simulink model "vc_coder"  (R2019b)
settings: Solver=FixedStepDiscrete  StartTime=0.0  StopTime=Inf  FixedStep=0.025  RelTol=1e-3  EnableMultiTasking=on
PreLoadFcn:
  | mdlname = bdroot;
  | oldFolder = cd(fileparts(which(mdlname)));
  | % cd ..\
  | 
  | load('./bus_type/bus_type.mat');
model workspace (MAT data in the model file):
  CLK = Simulink.Parameter
  CLK.Value = 200000000
  CLK.DataType = 'auto'
  CLK.Dimensions = [1 1]
  PWMFreq = Simulink.Parameter
  PWMFreq.Value = 1200
  PWMFreq.DataType = 'auto'
  PWMFreq.Dimensions = [1 1]
  RCDataLen = Simulink.Parameter
  RCDataLen.Value = 19
  RCDataLen.DataType = 'int8'
  RCDataLen.Dimensions = [1 1]
  StepSize = Simulink.Parameter
  StepSize.Value = 0.025
  StepSize.DataType = 'auto'
  StepSize.Dimensions = [1 1]
libraries: c2837xDlib x9, simulink x5, c280xlib x2, commutil2 x1, c2000lib x1
CloseFcn:
  | cd(oldFolder);
Description:
  | -> System Description <-
  | - Development environment:
  |     Matlab (version 2019b) with licence to
  |     - Simulink
  |     - Embedded Coder Support Package for Texas Instruments C2000 Processors
  |     - StateFlow
  | - Control board:
  |     TI LAUNCHXL F28379D
settings Model: SimulationMode=external  ExtModeTrigDuration=8  OrderedModelArguments=off  Creator=Quinn Ding  LastModifiedBy=Quinn
settings OptimizationCC: DefaultUnderspecifiedDataType=single  EnhancedBackFolding=on  PassReuseOutputArgsAs=Individual arguments  ZeroExternalMemoryAtStartup=off  MaxStackSize=1024  OptimizeBlockOrder=speed  DifferentSizesBufferReuse=on  OptimizationCustomize=off  DenormalBehavior=FlushToZero  EfficientTunableParamExpr=on
settings DebuggingCC: ParameterTunabilityLossMsg=error
settings HardwareCC: ProdBitPerChar=16  ProdBitPerInt=16  ProdBitPerPointer=32  ProdBitPerSizeT=32  ProdBitPerPtrDiffT=32  ProdLargestAtomicInteger=Integer  ProdLargestAtomicFloat=None  ProdWordSize=16  ProdLongLongMode=on  ProdHWDeviceType=Texas Instruments->C2000
settings SFSimCC: MATLABDynamicMemAlloc=off
settings RTWCC: SystemTargetFile=ert.tlc  HardwareBoard=TI Delfino F28379D LaunchPad  TLCOptions=-aInlineSetEventsForThisBaseRateFcn=TLC_FALSE -aSuppressMultiTaskScheduler=TLC_FALSE -aRateBasedStepFcn=1  TemplateMakefile=ert_default_tmf  Toolchain=Texas Instruments Code Composer Studio (C2000)  BuildConfiguration=Faster Runs  IncludeHyperlinkInReport=on
settings CodeAppCC: ForceParamTrailComments=on  IgnoreCustomStorageClasses=off  OperatorAnnotations=on  SimulinkDataObjDesc=on  SFDataObjDesc=on  InsertBlockDesc=on
settings ERTTargetCC: TargetLangStandard=C99 (ISO)  CodeReplacementLibrary=TI C28x  ExtModeStaticAllocSize=10000  RootIOFormat=Structure reference

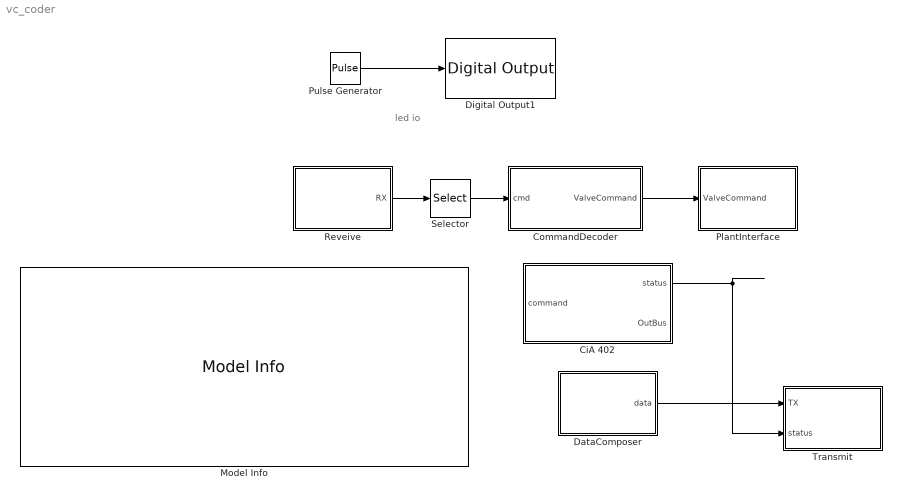
== system vc_coder ==
  note: led io
  CiA 402 : Stateflow chart  BlockKeywords=__PRM__SERIALIZED__DATA__:Stateflow Chart,Stateflow Diagram  TreatAsAtomicUnit=on
  CommandDecoder : Subsystem
  DataComposer : Subsystem
  Digital Output1 : c2837xDlib/Digital Output  GPIO_Number=GPIO24~GPIO31  GPIO_Bit0=off  GPIO_BIT0_Toggle=off  GPIO_Bit1=off  GPIO_BIT1_Toggle=off  GPIO_Bit2=off  GPIO_BIT2_Toggle=off  GPIO_Bit3=off  GPIO_BIT3_Toggle=off  GPIO_Bit4=off  GPIO_BIT4_Toggle=off  GPIO_Bit5=off  GPIO_BIT5_Toggle=off  GPIO_Bit6=off  GPIO_BIT6_Toggle=off  GPIO_Bit7=on  GPIO_BIT7_Toggle=off
      settings: SourceProductName=Embedded Coder Support Package for Texas Instruments C2000 Processors  SourceProductBaseCode=TIC2000
  Model Info : simulink/Model-Wide Utilities/Model Info  Frame=on  DisplayStringWithTags=|  HorizontalTextAlignment=Left  LeftAlignmentValue=0.02
      | DSP coder %<ModelVersion> of valve controller for the SMA actuator.
      | 
      | Developed by %<Creator> at the Surgical Robotics & Devices Laboratory, CUHK.
      | 
      | Last updated at %<LastModificationDate>.
      | 
      | %<Description>
  PlantInterface : Subsystem
  Pulse Generator : DiscretePulseGenerator  Period=100  PulseWidth=50  SampleTime=-1
  Reveive : Subsystem
  Selector : Selector  InputPortWidth=19  IndexOptions=Index vector (dialog)  Indices=[RCDataLen]  OutputSizes=1
  Transmit : Subsystem
  wires:
  Pulse Generator/1 -> Digital Output1/1
  CommandDecoder/1(ValveCommand) -> PlantInterface/1(ValveCommand)
  Reveive/1(RX) -> Selector/1
  DataComposer/1(data) -> Transmit/1(TX)
  CiA 402/1(status) -> Transmit/2(status)
  Selector/1 -> CommandDecoder/1(cmd)

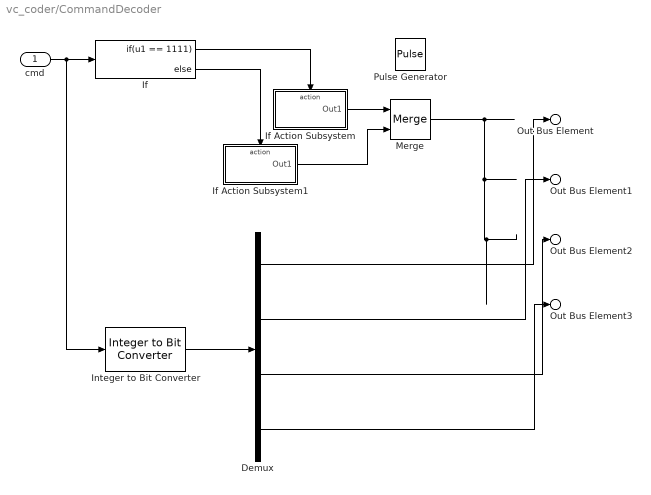
== system vc_coder/CommandDecoder ==
  cmd : Inport
  Demux : Demux
  If : If  IfExpression=u1 == 1111
  If Action Subsystem : Subsystem  TreatAsAtomicUnit=on
  If Action Subsystem1 : Subsystem  TreatAsAtomicUnit=on
  Integer to Bit Converter : commutil2/Integer to Bit Converter  nbits=4  signedInputValues=Unsigned  bitOrder=MSB first  outDtype=Inherit via internal rule
      settings: SourceProductName=Communications Toolbox
  Merge : Merge
  Pulse Generator : DiscretePulseGenerator  Period=80  PulseWidth=40  SampleTime=-1
  Out Bus Element : Outport  PortName=ValveCommand  Element=V1
  Out Bus Element1 : Outport  PortName=ValveCommand  Element=V2
  Out Bus Element2 : Outport  PortName=ValveCommand  Element=V3
  Out Bus Element3 : Outport  PortName=ValveCommand  Element=V4
  wires:
  Merge/1 -> ?
  If/1 -> If Action Subsystem/Action
  If/2 -> If Action Subsystem1/Action
  If Action Subsystem/1(Out1) -> Merge/1
  If Action Subsystem1/1(Out1) -> Merge/2
  cmd/1 -> Integer to Bit Converter/1, If/1
  Integer to Bit Converter/1 -> Demux/1
  Demux/1 -> Out Bus Element/1
  Demux/2 -> Out Bus Element1/1
  Demux/3 -> Out Bus Element2/1
  Demux/4 -> Out Bus Element3/1

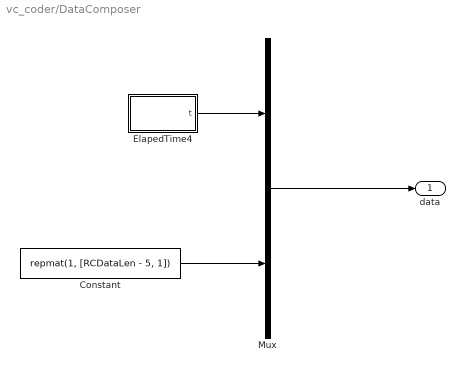
== system vc_coder/DataComposer ==
  Constant : Constant  Value=repmat(1, [RCDataLen - 5, 1])  OutDataTypeStr=single
  ElapedTime4 : Subsystem
  Mux : Mux  Inputs=2
  data : Outport
  wires:
  ElapedTime4/1(t) -> Mux/1
  Mux/1 -> data/1
  Constant/1 -> Mux/2

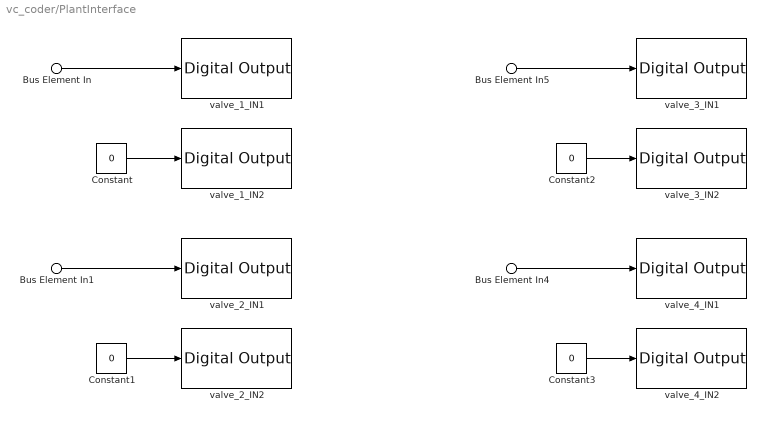
== system vc_coder/PlantInterface ==
  Bus Element In1 : Inport  PortName=ValveCommand  Element=V2
  Bus Element In : Inport  PortName=ValveCommand  Element=V1
  Bus Element In5 : Inport  PortName=ValveCommand  Element=V3
  Bus Element In4 : Inport  PortName=ValveCommand  Element=V4
  Constant{,1..3} (4 alike) : Constant  Value=0
  valve_1_IN1 : c2837xDlib/Digital Output  GPIO_Number=GPIO0~GPIO7  GPIO_Bit0=off  GPIO_BIT0_Toggle=off  GPIO_Bit1=off  GPIO_BIT1_Toggle=off  GPIO_Bit2=off  GPIO_BIT2_Toggle=off  GPIO_Bit3=off  GPIO_BIT3_Toggle=off  GPIO_Bit4=off  GPIO_BIT4_Toggle=off  GPIO_Bit5=off  GPIO_BIT5_Toggle=off  GPIO_Bit6=on  GPIO_BIT6_Toggle=off  GPIO_Bit7=off  GPIO_BIT7_Toggle=off
      settings: SourceProductName=Embedded Coder Support Package for Texas Instruments C2000 Processors  SourceProductBaseCode=TIC2000
  valve_1_IN2 : c2837xDlib/Digital Output  GPIO_Number=GPIO0~GPIO7  GPIO_Bit0=off  GPIO_BIT0_Toggle=off  GPIO_Bit1=off  GPIO_BIT1_Toggle=off  GPIO_Bit2=off  GPIO_BIT2_Toggle=off  GPIO_Bit3=off  GPIO_BIT3_Toggle=off  GPIO_Bit4=off  GPIO_BIT4_Toggle=off  GPIO_Bit5=off  GPIO_BIT5_Toggle=off  GPIO_Bit6=off  GPIO_BIT6_Toggle=off  GPIO_Bit7=on  GPIO_BIT7_Toggle=off
      settings: SourceProductName=Embedded Coder Support Package for Texas Instruments C2000 Processors  SourceProductBaseCode=TIC2000
  valve_2_IN1 : c2837xDlib/Digital Output  GPIO_Number=GPIO8~GPIO15  GPIO_Bit0=on  GPIO_BIT0_Toggle=off  GPIO_Bit1=off  GPIO_BIT1_Toggle=off  GPIO_Bit2=off  GPIO_BIT2_Toggle=off  GPIO_Bit3=off  GPIO_BIT3_Toggle=off  GPIO_Bit4=off  GPIO_BIT4_Toggle=off  GPIO_Bit5=off  GPIO_BIT5_Toggle=off  GPIO_Bit6=off  GPIO_BIT6_Toggle=off  GPIO_Bit7=off  GPIO_BIT7_Toggle=off
      settings: SourceProductName=Embedded Coder Support Package for Texas Instruments C2000 Processors  SourceProductBaseCode=TIC2000
  valve_2_IN2 : c2837xDlib/Digital Output  GPIO_Number=GPIO8~GPIO15  GPIO_Bit0=off  GPIO_BIT0_Toggle=off  GPIO_Bit1=on  GPIO_BIT1_Toggle=off  GPIO_Bit2=off  GPIO_BIT2_Toggle=off  GPIO_Bit3=off  GPIO_BIT3_Toggle=off  GPIO_Bit4=off  GPIO_BIT4_Toggle=off  GPIO_Bit5=off  GPIO_BIT5_Toggle=off  GPIO_Bit6=off  GPIO_BIT6_Toggle=off  GPIO_Bit7=off  GPIO_BIT7_Toggle=off
      settings: SourceProductName=Embedded Coder Support Package for Texas Instruments C2000 Processors  SourceProductBaseCode=TIC2000
  valve_3_IN1 : c2837xDlib/Digital Output  GPIO_Number=GPIO0~GPIO7  GPIO_Bit0=off  GPIO_BIT0_Toggle=off  GPIO_Bit1=off  GPIO_BIT1_Toggle=off  GPIO_Bit2=off  GPIO_BIT2_Toggle=off  GPIO_Bit3=off  GPIO_BIT3_Toggle=off  GPIO_Bit4=on  GPIO_BIT4_Toggle=off  GPIO_Bit5=off  GPIO_BIT5_Toggle=off  GPIO_Bit6=off  GPIO_BIT6_Toggle=off  GPIO_Bit7=off  GPIO_BIT7_Toggle=off
      settings: SourceProductName=Embedded Coder Support Package for Texas Instruments C2000 Processors  SourceProductBaseCode=TIC2000
  valve_3_IN2 : c2837xDlib/Digital Output  GPIO_Number=GPIO0~GPIO7  GPIO_Bit0=off  GPIO_BIT0_Toggle=off  GPIO_Bit1=off  GPIO_BIT1_Toggle=off  GPIO_Bit2=off  GPIO_BIT2_Toggle=off  GPIO_Bit3=off  GPIO_BIT3_Toggle=off  GPIO_Bit4=off  GPIO_BIT4_Toggle=off  GPIO_Bit5=on  GPIO_BIT5_Toggle=off  GPIO_Bit6=off  GPIO_BIT6_Toggle=off  GPIO_Bit7=off  GPIO_BIT7_Toggle=off
      settings: SourceProductName=Embedded Coder Support Package for Texas Instruments C2000 Processors  SourceProductBaseCode=TIC2000
  valve_4_IN1 : c2837xDlib/Digital Output  GPIO_Number=GPIO8~GPIO15  GPIO_Bit0=off  GPIO_BIT0_Toggle=off  GPIO_Bit1=off  GPIO_BIT1_Toggle=off  GPIO_Bit2=on  GPIO_BIT2_Toggle=off  GPIO_Bit3=off  GPIO_BIT3_Toggle=off  GPIO_Bit4=off  GPIO_BIT4_Toggle=off  GPIO_Bit5=off  GPIO_BIT5_Toggle=off  GPIO_Bit6=off  GPIO_BIT6_Toggle=off  GPIO_Bit7=off  GPIO_BIT7_Toggle=off
      settings: SourceProductName=Embedded Coder Support Package for Texas Instruments C2000 Processors  SourceProductBaseCode=TIC2000
  valve_4_IN2 : c2837xDlib/Digital Output  GPIO_Number=GPIO8~GPIO15  GPIO_Bit0=off  GPIO_BIT0_Toggle=off  GPIO_Bit1=off  GPIO_BIT1_Toggle=off  GPIO_Bit2=off  GPIO_BIT2_Toggle=off  GPIO_Bit3=on  GPIO_BIT3_Toggle=off  GPIO_Bit4=off  GPIO_BIT4_Toggle=off  GPIO_Bit5=off  GPIO_BIT5_Toggle=off  GPIO_Bit6=off  GPIO_BIT6_Toggle=off  GPIO_Bit7=off  GPIO_BIT7_Toggle=off
      settings: SourceProductName=Embedded Coder Support Package for Texas Instruments C2000 Processors  SourceProductBaseCode=TIC2000
  wires:
  Constant1/1 -> valve_2_IN2/1
  Bus Element In1/1 -> valve_2_IN1/1
  Constant/1 -> valve_1_IN2/1
  Bus Element In/1 -> valve_1_IN1/1
  Bus Element In5/1 -> valve_3_IN1/1
  Bus Element In4/1 -> valve_4_IN1/1
  Constant3/1 -> valve_4_IN2/1
  Constant2/1 -> valve_3_IN2/1

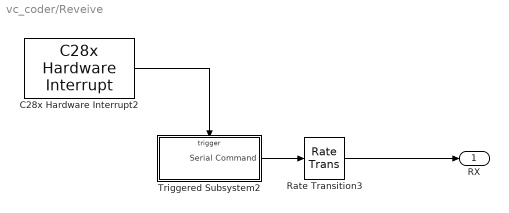
== system vc_coder/Reveive ==
  C28x Hardware Interrupt2 : c2000lib/Scheduling/C28x Hardware Interrupt  irqnumbers=[9]  pienumbers=[3]  irqpriorities=[30]  irqpreempts=[0]  showinput=off  dspchiptype=C280X
      settings: SourceProductName=Embedded Coder Support Package for Texas Instruments C2000 Processors  SourceProductBaseCode=TIC2000
  Rate Transition3 : RateTransition  Deterministic=off  OutPortSampleTimeOpt=Inherit
  Triggered Subsystem2 : Subsystem  TreatAsAtomicUnit=on
  RX : Outport
  wires:
  C28x Hardware Interrupt2/1 -> Triggered Subsystem2/Trigger
  Triggered Subsystem2/1(Serial Command) -> Rate Transition3/1
  Rate Transition3/1 -> RX/1

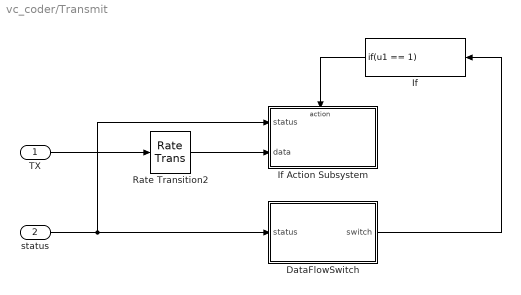
== system vc_coder/Transmit ==
  TX : Inport
  status : Inport  Port=2
  DataFlowSwitch : Subsystem
  If : If  IfExpression=u1 == 1  ShowElse=off
  If Action Subsystem : Subsystem  TreatAsAtomicUnit=on
  Rate Transition2 : RateTransition  Deterministic=off
  wires:
  If/1 -> If Action Subsystem/Action
  Rate Transition2/1 -> If Action Subsystem/2(data)
  TX/1 -> Rate Transition2/1
  status/1 -> If Action Subsystem/1(status), DataFlowSwitch/1(status)
  DataFlowSwitch/1(switch) -> If/1

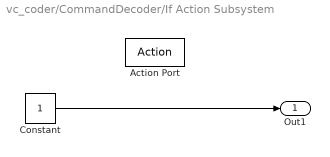
== system vc_coder/CommandDecoder/If Action Subsystem ==
  Action Port : ActionPort  ActionPortLabel=if(u1 == 1111)
  Constant : Constant
  Out1 : Outport
  wires:
  Constant/1 -> Out1/1

== system vc_coder/CommandDecoder/If Action Subsystem1 ==
  Action Port : ActionPort  ActionPortLabel=else
  Constant : Constant  Value=0
  Out1 : Outport
  wires:
  Constant/1 -> Out1/1

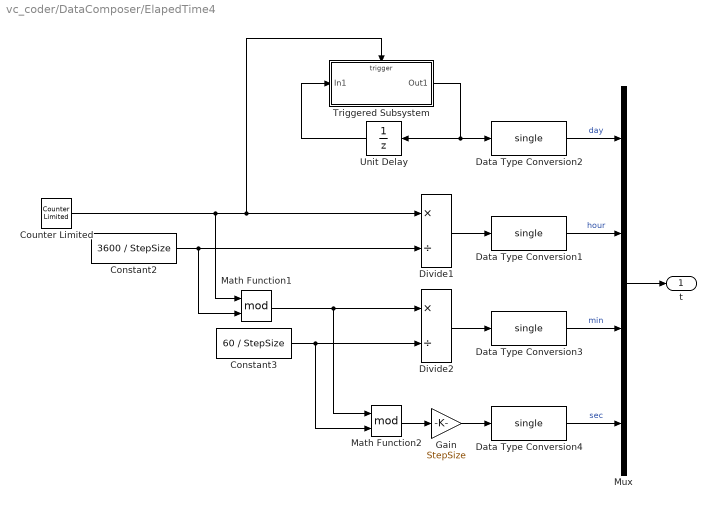
== system vc_coder/DataComposer/ElapedTime4 ==
  Constant2 : Constant  Value=3600 / StepSize  OutDataTypeStr=uint32
  Constant3 : Constant  Value=60 / StepSize  OutDataTypeStr=uint32
  Counter Limited : simulink/Sources/Counter Limited  uplimit=1 / StepSize * 60 * 60 * 24  tsamp=-1
  Data Type Conversion{1..4} (4 alike) : DataTypeConversion  OutDataTypeStr=single
  Divide1 : Product  Inputs=*/  OutDataTypeStr=uint8
  Divide2 : Product  Inputs=*/  OutDataTypeStr=uint8
  Gain : Gain  Gain=StepSize  OutDataTypeStr=single
  Math Function1 : Math  Operator=mod  SignedPower=off  SaturateOnIntegerOverflow=on
  Math Function2 : Math  Operator=mod  SignedPower=off  SaturateOnIntegerOverflow=on
  Mux : Mux
  Triggered Subsystem : Subsystem  TreatAsAtomicUnit=on
  Unit Delay : UnitDelay  SampleTime=-1  HasFrameUpgradeWarning=on
  t : Outport
  wires:
  Counter Limited/1 -> Divide1/1, Triggered Subsystem/Trigger, Math Function1/1
  Divide1/1 -> Data Type Conversion1/1
  Divide2/1 -> Data Type Conversion3/1
  Constant2/1 -> Math Function1/2, Divide1/2
  Math Function1/1 -> Divide2/1, Math Function2/1
  Data Type Conversion2/1 -> Mux/1  "day"
  Data Type Conversion1/1 -> Mux/2  "hour"
  Data Type Conversion3/1 -> Mux/3  "min"
  Data Type Conversion4/1 -> Mux/4  "sec"
  Math Function2/1 -> Gain/1
  Constant3/1 -> Divide2/2, Math Function2/2
  Mux/1 -> t/1
  Triggered Subsystem/1(Out1) -> Data Type Conversion2/1, Unit Delay/1
  Unit Delay/1 -> Triggered Subsystem/1(In1)
  Gain/1 -> Data Type Conversion4/1

== system vc_coder/Reveive/Triggered Subsystem2 ==
  SCIA RCV Interrupt : TriggerPort  TriggerType=function-call  VariantControl=Variant
  SCI Receive : c280xlib/SCI Receive  sciModule=B  dataHead=''  dataTail=''  dataType=single  dataDim=19  initValue=0  errOption=Output the last received value  errValue=0  sampleTime=-1  outputStatus=off  postInterrupt=on  numFifo=1
      settings: SourceProductName=Embedded Coder Support Package for Texas Instruments C2000 Processors  SourceProductBaseCode=TIC2000
  Serial Command : Outport
  wires:
  SCI Receive/1 -> Serial Command/1

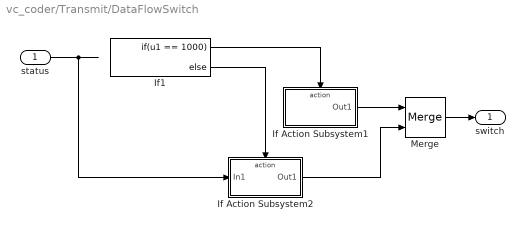
== system vc_coder/Transmit/DataFlowSwitch ==
  status : Inport
  If Action Subsystem1 : Subsystem  TreatAsAtomicUnit=on
  If Action Subsystem2 : Subsystem  TreatAsAtomicUnit=on
  If1 : If  IfExpression=u1 == 1000
  Merge : Merge
  switch : Outport
  wires:
  If Action Subsystem1/1(Out1) -> Merge/1
  If Action Subsystem2/1(Out1) -> Merge/2
  If1/2 -> If Action Subsystem2/Action
  Merge/1 -> switch/1
  If1/1 -> If Action Subsystem1/Action
  status/1 -> If Action Subsystem2/1(In1)

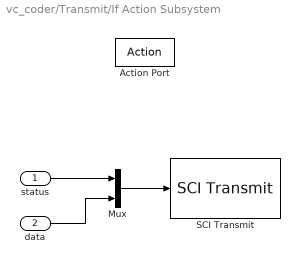
== system vc_coder/Transmit/If Action Subsystem ==
  status : Inport
  data : Inport  Port=2
  Action Port : ActionPort  ActionPortLabel=if(u1 == 1)
  Mux : Mux  Inputs=2
  SCI Transmit : c280xlib/SCI Transmit  sciModule=B  dataHead=''  dataTail=''  postInterrupt=off  numFifo=1
      settings: SourceProductName=Embedded Coder Support Package for Texas Instruments C2000 Processors
  wires:
  status/1 -> Mux/1
  data/1 -> Mux/2
  Mux/1 -> SCI Transmit/1

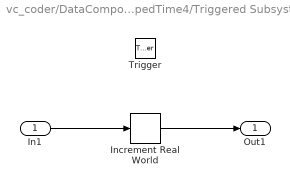
== system vc_coder/DataComposer/ElapedTime4/Triggered Subsystem ==
  In1 : Inport
  Trigger : TriggerPort  TriggerType=falling  VariantControl=Variant
  Increment Real World : simulink/Additional Math & Discrete/Additional Math: Increment - Decrement/Increment Real World
      settings: SourceProductName=Simulink  SourceProductBaseCode=SL
  Out1 : Outport
  wires:
  In1/1 -> Increment Real World/1
  Increment Real World/1 -> Out1/1

== system vc_coder/Transmit/DataFlowSwitch/If Action Subsystem1 ==
  Action Port : ActionPort  ActionPortLabel=if(u1 == 1000)
  Constant : Constant
  Out1 : Outport
  wires:
  Constant/1 -> Out1/1

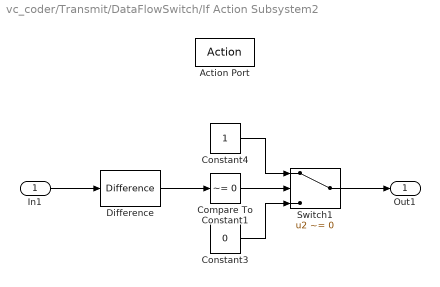
== system vc_coder/Transmit/DataFlowSwitch/If Action Subsystem2 ==
  In1 : Inport
  Action Port : ActionPort  ActionPortLabel=else
  Compare To Constant1 : simulink/Logic and Bit Operations/Compare To Constant  relop=~=  const=0  OutDataTypeStr=boolean
  Constant3 : Constant  Value=0
  Constant4 : Constant
  Difference : simulink/Discrete/Difference  ICPrevInput=0.0  OutMin=[]  OutMax=[]  OutDataType=fixdt(1, 16)  OutScaling=2^-10  DoSatur=off
  Switch1 : Switch  Criteria=u2 ~= 0
  Out1 : Outport
  wires:
  Switch1/1 -> Out1/1
  Compare To Constant1/1 -> Switch1/2
  In1/1 -> Difference/1
  Constant3/1 -> Switch1/3
  Difference/1 -> Compare To Constant1/1
  Constant4/1 -> Switch1/1

== stateflow chart vc_coder/CiA 402 ==
  state READY_TO_SWITCH_ON
    entry:
    status = 50;
    exit:
    ;
  state SWITCHED_ON
    entry:
    OutBus.EnableValve1 = 0;
    OutBus.EnableValve2 = 0;
    status = 51;
    exit:
    ;
  state OPERATION_ENABLE
    entry:
    OutBus.EnableValve1 = 1;
    OutBus.EnableValve2 = 1;
    status = 52;
    exit:
    ;
    state IDLE_MODE
      entry:
      status = 52;
    state PRECOOL_MODE
      entry:
      status = 53;
    (default) -> IDLE_MODE
    IDLE_MODE -> PRECOOL_MODE : [command(RCDataLen) == 14]
    PRECOOL_MODE -> IDLE_MODE : [command(RCDataLen) == 15]
  OPERATION_ENABLE -> READY_TO_SWITCH_ON [order 2] : [command(RCDataLen) == 0]
  SWITCHED_ON -> READY_TO_SWITCH_ON [order 3] : [command(RCDataLen) == 0]
  (default) -> READY_TO_SWITCH_ON
  SWITCHED_ON -> OPERATION_ENABLE [order 2] : [command(RCDataLen) == 12]
  READY_TO_SWITCH_ON -> SWITCHED_ON : [command(RCDataLen) == 10]
  SWITCHED_ON -> READY_TO_SWITCH_ON [order 1] : [command(RCDataLen) == 11]
  OPERATION_ENABLE -> SWITCHED_ON [order 1] : [command(RCDataLen) == 13]
  data: status output single; command input; OutBus output Bus: StateMachinOutBus; RCDataLen parameter
